simulink model "Task7"  (R2021b)
settings: Solver=VariableStepAuto  StartTime=0.0  StopTime=10.0  RelTol=1e-3
settings Model: Creator=mluser  LastModifiedBy=mluser

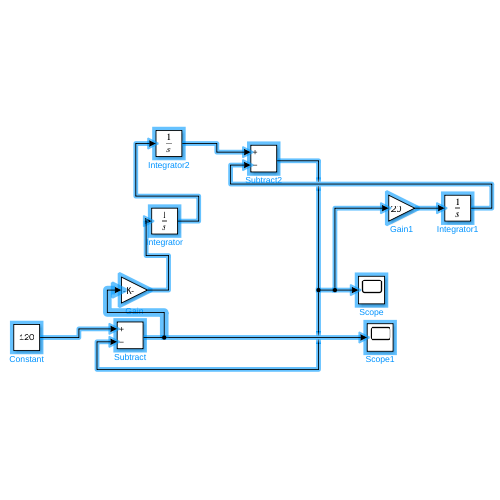
[thumbnail: Simulink's stored preview of the top-level diagram]
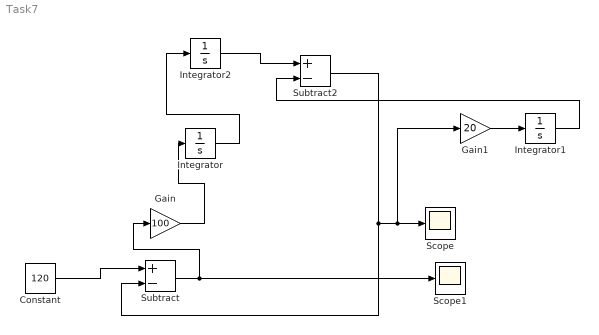
== system Task7 ==
  Constant : Constant  Value=120
  Gain : Gain  Gain=100
  Gain1 : Gain  Gain=20
  Integrator : Integrator
  Integrator1 : Integrator
  Integrator2 : Integrator
  Scope : Scope
  Scope1 : Scope
  Subtract : Sum  Inputs=+-
  Subtract2 : Sum  Inputs=+-
  wires:
  Integrator1/1 -> Subtract2/2
  Gain1/1 -> Integrator1/1
  Integrator/1 -> Integrator2/1
  Gain/1 -> Integrator/1
  Integrator2/1 -> Subtract2/1
  Constant/1 -> Subtract/1
  Subtract2/1 -> Subtract/2, Gain1/1, Scope/1
  Subtract/1 -> Gain/1, Scope1/1
